simulink model "riggs_iodine_model"  (R2018b)
settings: Solver=VariableStepAuto  StartTime=0.0  StopTime=400  RelTol=1e-3
libraries: simulink x3
settings Model: Creator=ASUS VivoBook  LastModifiedBy=ASUS VivoBook

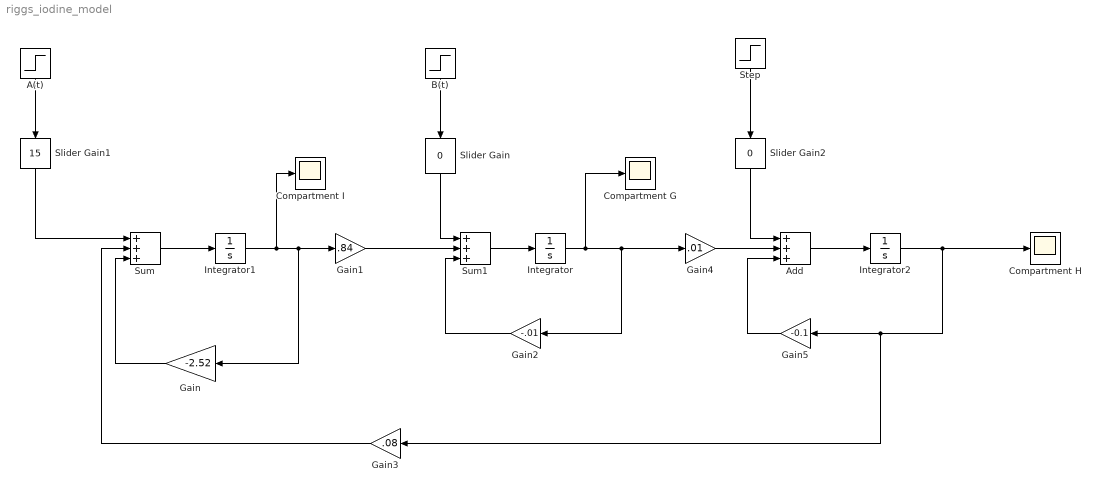
== system riggs_iodine_model ==
  A(t) : Step  SampleTime=0
  Add : Sum  Inputs=+++
  B(t) : Step  Time=0  SampleTime=0
  Compartment G : Scope
  Compartment H : Scope
  Compartment I : Scope
  Gain : Gain  Gain=-2.52
  Gain1 : Gain  Gain=.84
  Gain2 : Gain  Gain=-.01
  Gain3 : Gain  Gain=.08
  Gain4 : Gain  Gain=.01
  Gain5 : Gain  Gain=-0.1
  Integrator : Integrator  InitialCondition=6821
  Integrator1 : Integrator  InitialCondition=81
  Integrator2 : Integrator  InitialCondition=682
  Slider Gain : simulink/Math Operations/Slider Gain  gain=0  low=0  high=2
  Slider Gain1 : simulink/Math Operations/Slider Gain  gain=15  low=0  high=20
  Slider Gain2 : simulink/Math Operations/Slider Gain  gain=0  low=0  high=2
  Step : Step  SampleTime=0
  Sum : Sum  Inputs=+++
  Sum1 : Sum  Inputs=+++
  wires:
  A(t)/1 -> Slider Gain1/1
  Slider Gain1/1 -> Sum/1
  Sum/1 -> Integrator1/1
  Integrator1/1 -> Compartment I/1, Gain1/1, Gain/1
  Gain/1 -> Sum/3
  Gain1/1 -> Sum1/2
  Slider Gain/1 -> Sum1/1
  B(t)/1 -> Slider Gain/1
  Sum1/1 -> Integrator/1
  Integrator/1 -> Compartment G/1, Gain4/1, Gain2/1
  Gain2/1 -> Sum1/3
  Gain3/1 -> Sum/2
  Gain4/1 -> Add/2
  Slider Gain2/1 -> Add/1
  Step/1 -> Slider Gain2/1
  Gain5/1 -> Add/3
  Add/1 -> Integrator2/1
  Integrator2/1 -> Gain5/1, Gain3/1, Compartment H/1
